simulink model "Modelo_LTI_equivalente_aum"  (R2017a)
settings: Solver=VariableStepAuto  StartTime=0.0  StopTime=1  MaxStep=1e-4  RelTol=1e-3
values from neighbouring files (symbols this model uses):
  beq = bl/r^2 + bm    (= 1.5638971155e-05)    [Evaluacion_polos_5_2_2.m]    (also in modelo_global_NL.m = 1.5e-05)
  Jeq = Jl/r^2 + Jm    (= 6.9338269301e-06)    [Evaluacion_polos_5_2_2.m]    (also in modelo_global_NL.m = 5.65588462007e-06)
  LambdaM = 0.01546    [Evaluacion_polos_5_2_2.m]    (also in modelo_global_NL.m)
  Ld = 0.0066    [Evaluacion_polos_5_2_2.m]    (also in modelo_global_NL.m)
  Lq = 0.0058    [Evaluacion_polos_5_2_2.m]    (also in modelo_global_NL.m)
  Pp = 3    [Evaluacion_polos_5_2_2.m]    (also in modelo_global_NL.m)
  Rs = 1.02    [Evaluacion_polos_5_2_2.m]    (also in modelo_global_NL.m)
undefined symbols (not defined in the file or in its folder): sigbuilder_block
settings Model: Creator=merem  LastModifiedBy=merem

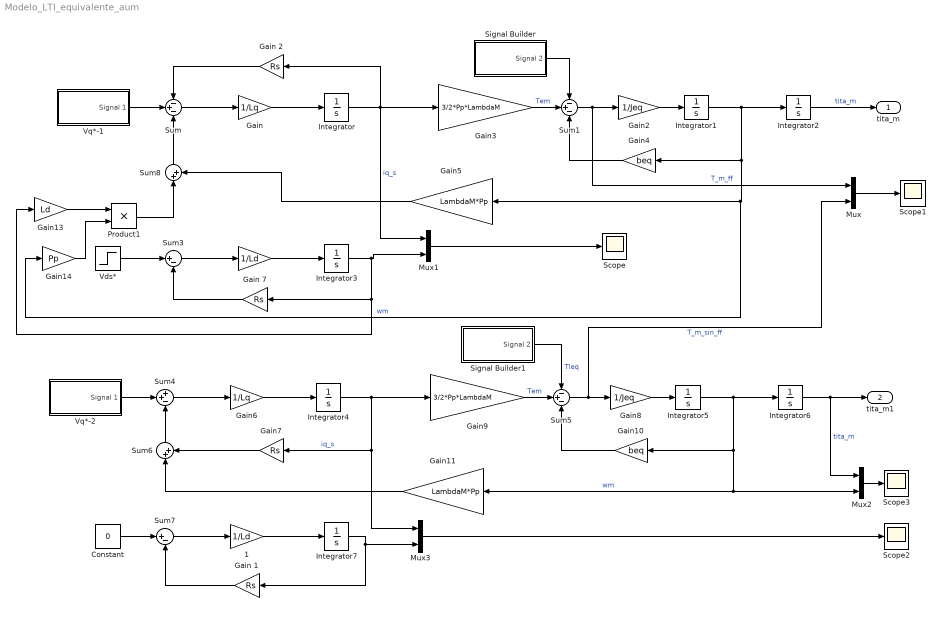
== system Modelo_LTI_equivalente_aum ==
  " " : Gain  Gain=1/Ld
  " 1" : Gain  Gain=1/Ld
  Constant : Constant  Value=0
  Gain : Gain  Gain=1/Lq
  Gain 1 : Gain  Gain=Rs
  Gain 2 : Gain  Gain=Rs
  Gain 7 : Gain  Gain=Rs
  Gain10 : Gain  Gain=beq
  Gain11 : Gain  Gain=LambdaM*Pp
  Gain13 : Gain  Gain=Ld
  Gain14 : Gain  Gain=Pp
  Gain2 : Gain  Gain=1/Jeq
  Gain3 : Gain  Gain=3/2*Pp*LambdaM
  Gain4 : Gain  Gain=beq
  Gain5 : Gain  Gain=LambdaM*Pp
  Gain6 : Gain  Gain=1/Lq
  Gain7 : Gain  Gain=Rs
  Gain8 : Gain  Gain=1/Jeq
  Gain9 : Gain  Gain=3/2*Pp*LambdaM
  Integrator{,1..7} (8 alike) : Integrator
  Mux{,1..3} (4 alike) : Mux  Inputs=2
  Product1 : Product
  Scope{,1..3} (4 alike) : Scope
  Signal Builder : Subsystem  Tag=STV Subsys  LoadFcn=sigbuilder_block('load');  StartFcn=sigbuilder_block('start');  StopFcn=sigbuilder_block('stop');  ClipboardFcn=sigbuilder_block('clipboard');  mask(Sigbuilder block){tuvar=[0:10]}
      mask help: Simulink:masks:SigbuilderBlock_MD
      mask init:
      | if ~strcmp(get_param(bdroot(gcbh),'SimulationStatus'),'stopped') tuvar = sigbuilder_block('maskInit'); end
      settings: CopyFcn=sigbuilder_block('copy');  DeleteFcn=sigbuilder_block('delete');  ModelCloseFcn=sigbuilder_block('modelClose');  PreSaveFcn=sigbuilder_block('preSave');  PauseFcn=sigbuilder_block('pause');  ContinueFcn=sigbuilder_block('continue');  NameChangeFcn=sigbuilder_block('namechange');  OpenFcn=sigbuilder_block('open',[6 30 1012.5 447.75 ]);  CloseFcn=sigbuilder_block('close');
      mask Display: plot(0, 0, 100, 100,[2, 2, 32, 32, 2], [68, 8, 8, 68, 68],[32, 2], [38, 38], [32, 19, 2],[53, 60, 44], [32, 17, 17, 2],[16, 16, 31, 31]);txt = getActiveGroup(gcbh);text(2, 100, txt,'verticalAlignment', 'top');
  Signal Builder1 : Subsystem  Tag=STV Subsys  LoadFcn=sigbuilder_block('load');  StartFcn=sigbuilder_block('start');  StopFcn=sigbuilder_block('stop');  ClipboardFcn=sigbuilder_block('clipboard');  mask(Sigbuilder block){tuvar=[0:10]}
      mask help: Simulink:masks:SigbuilderBlock_MD
      mask init:
      | if ~strcmp(get_param(bdroot(gcbh),'SimulationStatus'),'stopped') tuvar = sigbuilder_block('maskInit'); end
      settings: CopyFcn=sigbuilder_block('copy');  DeleteFcn=sigbuilder_block('delete');  ModelCloseFcn=sigbuilder_block('modelClose');  PreSaveFcn=sigbuilder_block('preSave');  PauseFcn=sigbuilder_block('pause');  ContinueFcn=sigbuilder_block('continue');  NameChangeFcn=sigbuilder_block('namechange');  OpenFcn=sigbuilder_block('open',[6 30 1012.5 447.75 ]);  CloseFcn=sigbuilder_block('close');
      mask Display: plot(0, 0, 100, 100,[2, 2, 32, 32, 2], [68, 8, 8, 68, 68],[32, 2], [38, 38], [32, 19, 2],[53, 60, 44], [32, 17, 17, 2],[16, 16, 31, 31]);txt = getActiveGroup(gcbh);text(2, 100, txt,'verticalAlignment', 'top');
  Sum : Sum  Inputs=-+-
  Sum1 : Sum  Inputs=-+-
  Sum3 : Sum  Inputs=|+-
  Sum4 : Sum  Inputs=++-
  Sum5 : Sum  Inputs=-+-
  Sum6 : Sum  Inputs=|++
  Sum7 : Sum  Inputs=|+-
  Sum8 : Sum  Inputs=|++
  Vds* : Step  Time=0.5  After=1.9596  SampleTime=0
  Vq*-1 : Subsystem  Tag=STV Subsys  LoadFcn=sigbuilder_block('load');  StartFcn=sigbuilder_block('start');  StopFcn=sigbuilder_block('stop');  ClipboardFcn=sigbuilder_block('clipboard');  mask(Sigbuilder block){tuvar=[0:10]}
      mask help: Simulink:masks:SigbuilderBlock_MD
      mask init:
      | if ~strcmp(get_param(bdroot(gcbh),'SimulationStatus'),'stopped') tuvar = sigbuilder_block('maskInit'); end
      settings: CopyFcn=sigbuilder_block('copy');  DeleteFcn=sigbuilder_block('delete');  ModelCloseFcn=sigbuilder_block('modelClose');  PreSaveFcn=sigbuilder_block('preSave');  PauseFcn=sigbuilder_block('pause');  ContinueFcn=sigbuilder_block('continue');  NameChangeFcn=sigbuilder_block('namechange');  OpenFcn=sigbuilder_block('open',[6 -3.75 1012.5 407.25 ]);  CloseFcn=sigbuilder_block('close');
      mask Display: plot(0, 0, 100, 100,[2, 2, 32, 32, 2], [68, 8, 8, 68, 68],[32, 2], [38, 38], [32, 19, 2],[53, 60, 44], [32, 17, 17, 2],[16, 16, 31, 31]);txt = getActiveGroup(gcbh);text(2, 100, txt,'verticalAlignment', 'top');
  Vq*-2 : Subsystem  Tag=STV Subsys  LoadFcn=sigbuilder_block('load');  StartFcn=sigbuilder_block('start');  StopFcn=sigbuilder_block('stop');  ClipboardFcn=sigbuilder_block('clipboard');  mask(Sigbuilder block){tuvar=[0:10]}
      mask help: Simulink:masks:SigbuilderBlock_MD
      mask init:
      | if ~strcmp(get_param(bdroot(gcbh),'SimulationStatus'),'stopped') tuvar = sigbuilder_block('maskInit'); end
      settings: CopyFcn=sigbuilder_block('copy');  DeleteFcn=sigbuilder_block('delete');  ModelCloseFcn=sigbuilder_block('modelClose');  PreSaveFcn=sigbuilder_block('preSave');  PauseFcn=sigbuilder_block('pause');  ContinueFcn=sigbuilder_block('continue');  NameChangeFcn=sigbuilder_block('namechange');  OpenFcn=sigbuilder_block('open',[6 -3.75 1012.5 407.25 ]);  CloseFcn=sigbuilder_block('close');
      mask Display: plot(0, 0, 100, 100,[2, 2, 32, 32, 2], [68, 8, 8, 68, 68],[32, 2], [38, 38], [32, 19, 2],[53, 60, 44], [32, 17, 17, 2],[16, 16, 31, 31]);txt = getActiveGroup(gcbh);text(2, 100, txt,'verticalAlignment', 'top');
  tita_m : Outport
  tita_m1 : Outport  Port=2
  wires:
  Sum/1 -> Gain/1
  Gain/1 -> Integrator/1
  Integrator/1 -> Gain 2/1, Mux1/1, Gain3/1  "iq_s"
  Sum1/1 -> Mux/1, Gain2/1  "T_m_ff"
  Gain2/1 -> Integrator1/1
  Integrator1/1 -> Integrator2/1, Gain14/1, Gain5/1, Gain4/1  "wm"
  Integrator2/1 -> tita_m/1  "tita_m"
  Gain4/1 -> Sum1/3
  Gain3/1 -> Sum1/2  "Tem"
  " "/1 -> Integrator3/1
  Integrator3/1 -> Mux1/2, Gain13/1, Gain 7/1
  Gain 7/1 -> Sum3/2
  Mux/1 -> Scope1/1
  Mux1/1 -> Scope/1
  Vds*/1 -> Sum3/1
  Mux2/1 -> Scope3/1
  Sum4/1 -> Gain6/1
  Mux3/1 -> Scope2/1
  Sum7/1 -> " 1"/1
  Integrator5/1 -> Integrator6/1, Mux2/2, Gain11/1, Gain10/1  "wm"
  " 1"/1 -> Integrator7/1
  Signal Builder1/1(Signal 2) -> Sum5/1  "Tleq"
  Gain9/1 -> Sum5/2  "Tem"
  Gain 1/1 -> Sum7/2
  Gain8/1 -> Integrator5/1
  Gain7/1 -> Sum6/2
  Integrator6/1 -> Mux2/1, tita_m1/1  "tita_m"
  Gain11/1 -> Sum6/1
  Gain10/1 -> Sum5/3
  Integrator4/1 -> Mux3/1, Gain7/1, Gain9/1  "iq_s"
  Sum5/1 -> Mux/2, Gain8/1  "T_m_sin_ff"
  Gain6/1 -> Integrator4/1
  Signal Builder/1(Signal 2) -> Sum1/1
  Constant/1 -> Sum7/1
  Sum6/1 -> Sum4/3
  Vq*-2/1(Signal 1) -> Sum4/2
  Integrator7/1 -> Gain 1/1, Mux3/2
  Gain13/1 -> Product1/1
  Gain14/1 -> Product1/2
  Product1/1 -> Sum8/1
  Gain5/1 -> Sum8/2
  Sum3/1 -> " "/1
  Vq*-1/1(Signal 1) -> Sum/2
  Sum8/1 -> Sum/3
  Gain 2/1 -> Sum/1

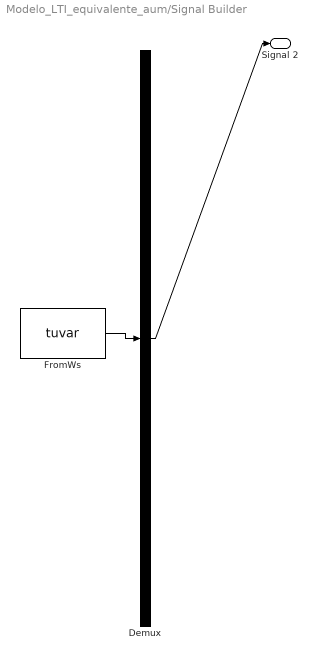
== system Modelo_LTI_equivalente_aum/Signal Builder ==
  Demux : Demux  Tag=STV Demux  Outputs=1
  FromWs : FromWorkspace  Tag=STV FromWs  VariableName=tuvar  SampleTime=0
      SigBuilderData=|
      | common.afterFinalStr = 'Extrapolate'
      | common.sampleTime = 0
      | dataSet.timeRange = [0 2]
      | dataSet.name = 'Group 1'
      | sbobj.Groups.Name = 'Group 1'
      | sbobj.Groups.Signals.Name = 'Signal 2'
      | sbobj.Groups.Signals.XData = [0 0.3 0.3 0.5 0.5 0.9 0.9 2]
      | sbobj.Groups.Signals.YData = [0 0 0.02 0.02 -0.02 -0.02 0 0]
      | sbobj.Groups.TimeRange = [0 2]
  Signal 2 : Outport  Tag=STV Outport
  wires:
  FromWs/1 -> Demux/1
  Demux/1 -> Signal 2/1

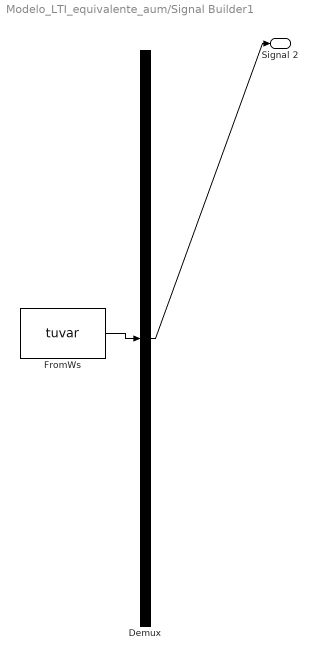
== system Modelo_LTI_equivalente_aum/Signal Builder1 ==
  Demux : Demux  Tag=STV Demux  Outputs=1
  FromWs : FromWorkspace  Tag=STV FromWs  VariableName=tuvar  SampleTime=0
      SigBuilderData=|
      | common.afterFinalStr = 'Extrapolate'
      | common.sampleTime = 0
      | dataSet.timeRange = [0 2]
      | dataSet.name = 'Group 1'
      | sbobj.Groups.Name = 'Group 1'
      | sbobj.Groups.Signals.Name = 'Signal 2'
      | sbobj.Groups.Signals.XData = [0 0.3 0.3 0.5 0.5 0.9 0.9 2]
      | sbobj.Groups.Signals.YData = [0 0 0.02 0.02 -0.02 -0.02 0 0]
      | sbobj.Groups.TimeRange = [0 2]
  Signal 2 : Outport  Tag=STV Outport
  wires:
  FromWs/1 -> Demux/1
  Demux/1 -> Signal 2/1

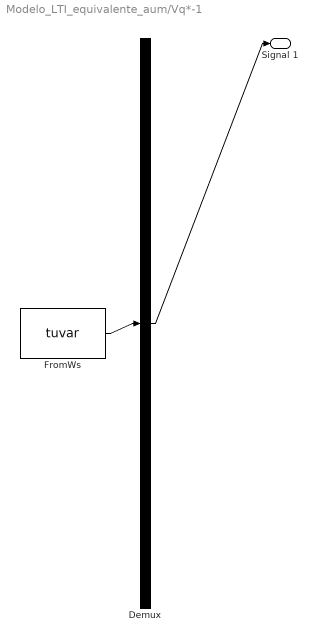
== system Modelo_LTI_equivalente_aum/Vq*-1 ==
  Demux : Demux  Tag=STV Demux  Outputs=1
  FromWs : FromWorkspace  Tag=STV FromWs  VariableName=tuvar  SampleTime=0
      SigBuilderData=|
      | common.afterFinalStr = 'Extrapolate'
      | common.sampleTime = 0
      | dataSet.timeRange = [0 2]
      | dataSet.name = 'Group 1'
      | sbobj.Groups.Name = 'Group 1'
      | sbobj.Groups.Signals.Name = 'Signal 1'
      | sbobj.Groups.Signals.XData = [0 0.096 0.096 0.7 0.7 2]
      | sbobj.Groups.Signals.YData = [0 0 19.56 19.56 0 0]
      | sbobj.Groups.TimeRange = [0 2]
  Signal 1 : Outport  Tag=STV Outport
  wires:
  Demux/1 -> Signal 1/1
  FromWs/1 -> Demux/1

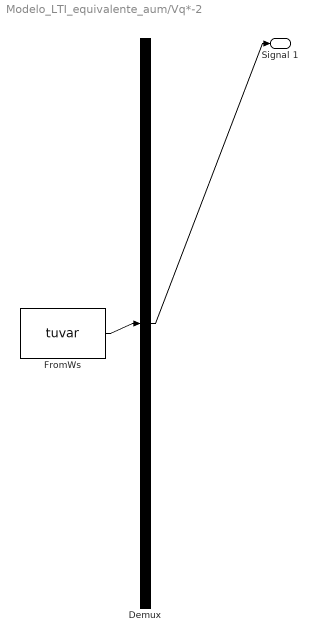
== system Modelo_LTI_equivalente_aum/Vq*-2 ==
  Demux : Demux  Tag=STV Demux  Outputs=1
  FromWs : FromWorkspace  Tag=STV FromWs  VariableName=tuvar  SampleTime=0
      SigBuilderData=|
      | common.afterFinalStr = 'Extrapolate'
      | common.sampleTime = 0
      | dataSet.timeRange = [0 2]
      | dataSet.name = 'Group 1'
      | sbobj.Groups.Name = 'Group 1'
      | sbobj.Groups.Signals.Name = 'Signal 1'
      | sbobj.Groups.Signals.XData = [0 0.096 0.096 0.7 0.7 2]
      | sbobj.Groups.Signals.YData = [0 0 19.56 19.56 0 0]
      | sbobj.Groups.TimeRange = [0 2]
  Signal 1 : Outport  Tag=STV Outport
  wires:
  Demux/1 -> Signal 1/1
  FromWs/1 -> Demux/1
